simulink model "DAC"  (R2023a)
settings: Solver=VariableStepAuto  StartTime=0.0  StopTime=10.0  RelTol=1e-3
libraries: dspsigops x1
settings Model: Creator=Алексей  LastModifiedBy=Алексей

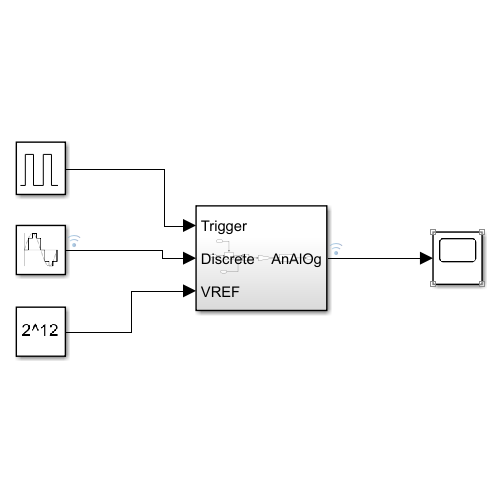
[thumbnail: Simulink's stored preview of the top-level diagram]
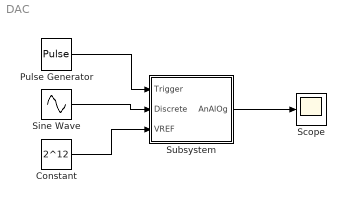
== system DAC ==
  Constant : Constant  Value=2^12
  Pulse Generator : DiscretePulseGenerator  PulseType=Time based  Period=0.1  PulseWidth=0.02
  Scope : Scope
  Sine Wave : Sin  SampleTime=0.1
  Subsystem : Subsystem
  wires:
  Sine Wave/1 -> Subsystem/2(Discrete)
  Constant/1 -> Subsystem/3(VREF)
  Subsystem/1(AnAlOg) -> Scope/1
  Pulse Generator/1 -> Subsystem/1(Trigger)

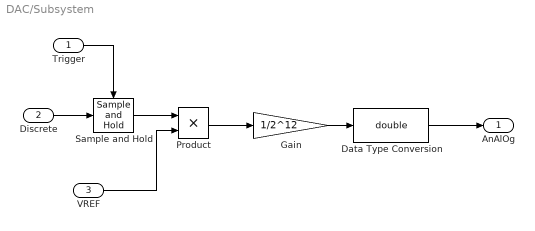
== system DAC/Subsystem ==
  Trigger : Inport
  Discrete : Inport  Port=2
  VREF : Inport  Port=3
  Data Type Conversion : DataTypeConversion  OutDataTypeStr=double  SaturateOnIntegerOverflow=off  RndMeth=Floor
  Gain : Gain  Gain=1/2^12
  Product : Product
  Sample and Hold : dspsigops/Sample and Hold  trig=Rising edge  initCond=0  latchinput=off
  AnAlOg : Outport
  wires:
  Gain/1 -> Data Type Conversion/1
  Product/1 -> Gain/1
  Sample and Hold/1 -> Product/1
  Trigger/1 -> Sample and Hold/Trigger
  VREF/1 -> Product/2
  Discrete/1 -> Sample and Hold/1
  Data Type Conversion/1 -> AnAlOg/1
